simulink model "SSGraph"  (R2020a)
settings: Solver=ode4  StartTime=0.0  StopTime=10  FixedStep=1e-3  RelTol=1e-3  EnableMultiTasking=on
values from neighbouring files (symbols this model uses):
  a = [-1 0 -1;-2 2 0;-1 0 -1]    [Espacio_d_Estados.m]    (also in dinam19.m = 2; examSisDin.m = [1 0 -1;2 0 1;1 0 3])
  b = [1 2 0]'    [Espacio_d_Estados.m]
settings Model: Creator=HP  LastModifiedBy=megat
settings DataIOCC: LimitDataPoints=on  SaveFormat=Array  ReturnWorkspaceOutputs=off
settings OptimizationCC: LifeSpan=inf
settings DebuggingCC: SFUnexpectedBacktrackingDiag=warning  SFNoUnconditionalDefaultTransitionDiag=warning  SFExecutionAtInitializationDiag=none  ArithmeticOperatorsInVariantConditions=warning
settings HardwareCC: ProdBitPerPointer=32  ProdBitPerSizeT=32  ProdBitPerPtrDiffT=32  ProdLargestAtomicFloat=None  ProdIntDivRoundTo=Undefined  ProdEndianess=Unspecified  ProdWordSize=32  ProdHWDeviceType=32-bit Generic
settings ModelReferenceCC: PropagateSignalLabelsOutOfModel=off
settings SFSimCC: SimUseLocalCustomCode=off  CustomCodeUndefinedFunction=UseInterfaceOnly
settings RTWCC: RTWUseLocalCustomCode=off
settings CodeAppCC: StateflowObjectComments=on
settings GRTTargetCC: TargetLangStandard=C89/C90 (ANSI)
settings ConfigComp: CovMetricSettings=dw  CovHtmlReporting=on  CovSaveCumulativeToWorkspaceVar=on  CovSaveSingleToWorkspaceVar=on  CovExternalEMLEnable=off

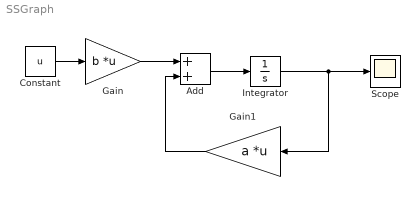
== system SSGraph ==
  Add : Sum
  Constant : Constant  Value=u
  Gain : Gain  Gain=b  Multiplication=Matrix(K*u)
  Gain1 : Gain  Gain=a  Multiplication=Matrix(K*u)
  Integrator : Integrator  InitialCondition=[0 0]
  Scope : Scope
  wires:
  Add/1 -> Integrator/1
  Constant/1 -> Gain/1
  Gain/1 -> Add/1
  Gain1/1 -> Add/2
  Integrator/1 -> Scope/1, Gain1/1
